simulink model "chains"  (R2025a)
settings: Solver=VariableStepAuto  StartTime=0.0  StopTime=20  RelTol=1e-3
libraries: dspsrcs4 x1
settings Model: Creator=konstantin  LastModifiedBy=konstantin

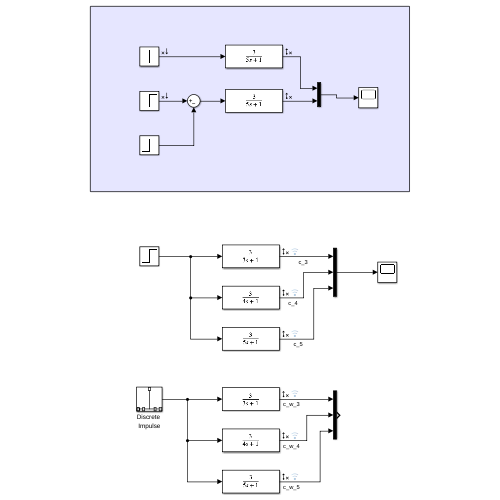
[thumbnail: Simulink's stored preview of the top-level diagram]
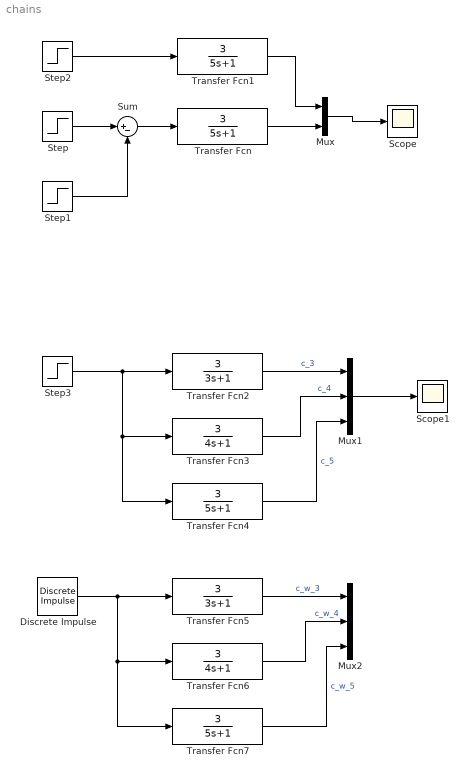
== system chains ==
  Discrete Impulse : dspsrcs4/Discrete  Impulse  Delay=0  SampleTime=1  FrameSample=1  OutputFrames=off  dataType=double  isSigned=on  wordLen=16  udDataType=sfix(16)  fracBitsMode=Best precision  numFracBits=15  OutDataTypeStr=double  LastOutDataTypeStr=double
  Mux : Mux  Inputs=2
  Mux1 : Mux  Inputs=3
  Mux2 : Mux  Inputs=3
  Scope : Scope
      settings: ActiveDisplayYMinimum=-0.31301291691381672  ActiveDisplayYMaximum=2.8171162522243511
  Scope1 : Scope
      settings: ActiveDisplayYMinimum=-1  ActiveDisplayYMaximum=1
  Step : Step  After=100  SampleTime=0
  Step1 : Step  Time=1.01  After=100  SampleTime=0
  Step2 : Step  SampleTime=0
  Step3 : Step  SampleTime=0
  Sum : Sum  Inputs=|+-
  Transfer Fcn{,1,4,7} (4 alike) : TransferFcn  Numerator=[3]  Denominator=[5 1]
  Transfer Fcn2 : TransferFcn  Numerator=[3]  Denominator=[3 1]
  Transfer Fcn3 : TransferFcn  Numerator=[3]  Denominator=[4 1]
  Transfer Fcn5 : TransferFcn  Numerator=[3]  Denominator=[3 1]
  Transfer Fcn6 : TransferFcn  Numerator=[3]  Denominator=[4 1]
  wires:
  Step/1 -> Sum/1
  Sum/1 -> Transfer Fcn/1
  Step1/1 -> Sum/2
  Transfer Fcn/1 -> Mux/2
  Mux/1 -> Scope/1
  Step2/1 -> Transfer Fcn1/1
  Transfer Fcn1/1 -> Mux/1
  Step3/1 -> Transfer Fcn4/1, Transfer Fcn3/1, Transfer Fcn2/1
  Transfer Fcn2/1 -> Mux1/1  "c_3"
  Transfer Fcn3/1 -> Mux1/2  "c_4"
  Transfer Fcn4/1 -> Mux1/3  "c_5"
  Mux1/1 -> Scope1/1
  Discrete Impulse/1 -> Transfer Fcn7/1, Transfer Fcn6/1, Transfer Fcn5/1
  Transfer Fcn5/1 -> Mux2/1  "c_w_3"
  Transfer Fcn6/1 -> Mux2/2  "c_w_4"
  Transfer Fcn7/1 -> Mux2/3  "c_w_5"
